simulink model "mechat_taklif2"  (R2016a)
settings: Solver=ode1  StartTime=0.0  StopTime=10.0  FixedStep=0.01  RelTol=1e-3
settings Model: Creator=ALA  LastModifiedBy=ALA

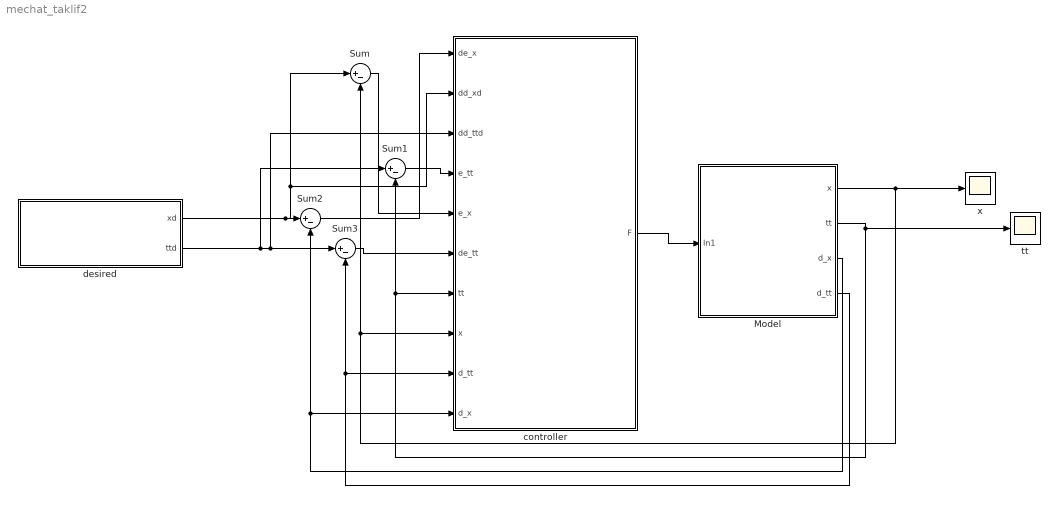
== system mechat_taklif2 ==
  Model : Subsystem
  Sum{,1..3} (4 alike) : Sum  Inputs=|+-
  controller : Subsystem
  desired : Subsystem
  tt : Scope
  x : Scope
  wires:
  controller/1(F) -> Model/1(In1)
  Model/1(x) -> Sum/2, controller/8(x), x/1
  desired/1(xd) -> controller/2(dd_xd), Sum/1, Sum2/1
  desired/2(ttd) -> controller/3(dd_ttd), Sum3/1, Sum1/1
  Model/4(d_tt) -> Sum3/2, controller/9(d_tt)
  Sum/1 -> controller/5("e_x ")
  Sum1/1 -> controller/4("e_tt ")
  Sum2/1 -> controller/1(de_x)
  Sum3/1 -> controller/6(de_tt)
  Model/2(tt) -> Sum1/2, controller/7("tt "), tt/1
  Model/3(d_x) -> Sum2/2, controller/10(d_x)

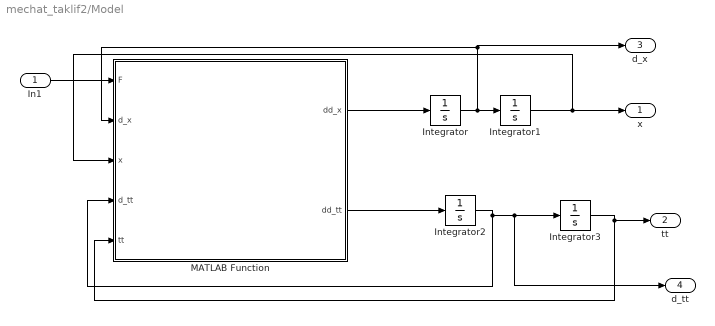
== system mechat_taklif2/Model ==
  In1 : Inport
  Integrator : Integrator
  Integrator1 : Integrator
  Integrator2 : Integrator
  Integrator3 : Integrator  InitialCondition=0.1
  MATLAB Function : MATLAB Function  TreatAsAtomicUnit=on
  x : Outport
  tt : Outport  Port=2
  d_x : Outport  Port=3
  d_tt : Outport  Port=4
  wires:
  In1/1 -> MATLAB Function/1(F)
  MATLAB Function/1(dd_x) -> Integrator/1
  Integrator/1 -> d_x/1, MATLAB Function/2(d_x), Integrator1/1
  Integrator1/1 -> x/1, MATLAB Function/3(x)
  Integrator2/1 -> MATLAB Function/4(d_tt), d_tt/1, Integrator3/1
  Integrator3/1 -> tt/1, MATLAB Function/5(tt)
  MATLAB Function/2(dd_tt) -> Integrator2/1

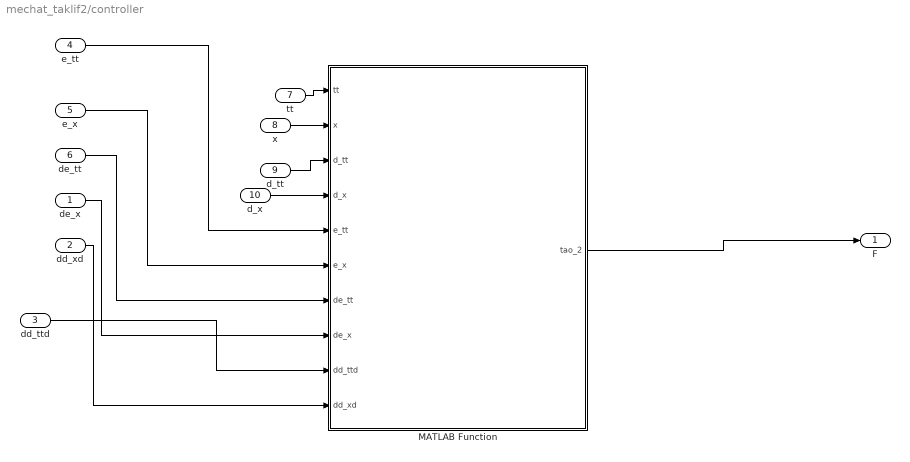
== system mechat_taklif2/controller ==
  de_x : Inport
  dd_xd : Inport  Port=2
  dd_ttd : Inport  Port=3
  "e_tt " : Inport  Port=4
  "e_x " : Inport  Port=5
  de_tt : Inport  Port=6
  "tt " : Inport  Port=7
  x : Inport  Port=8
  d_tt : Inport  Port=9
  d_x : Inport  Port=10
  MATLAB Function : MATLAB Function  TreatAsAtomicUnit=on
  F : Outport
  wires:
  "e_tt "/1 -> MATLAB Function/5(e_tt)
  "e_x "/1 -> MATLAB Function/6(e_x)
  de_tt/1 -> MATLAB Function/7(de_tt)
  de_x/1 -> MATLAB Function/8(de_x)
  dd_xd/1 -> MATLAB Function/10(dd_xd)
  dd_ttd/1 -> MATLAB Function/9(dd_ttd)
  "tt "/1 -> MATLAB Function/1(tt)
  x/1 -> MATLAB Function/2(x)
  d_tt/1 -> MATLAB Function/3(d_tt)
  d_x/1 -> MATLAB Function/4(d_x)
  MATLAB Function/1(tao_2) -> F/1

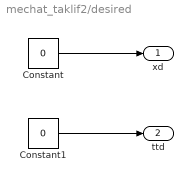
== system mechat_taklif2/desired ==
  Constant : Constant  Value=0
  Constant1 : Constant  Value=0
  xd : Outport
  ttd : Outport  Port=2
  wires:
  Constant/1 -> xd/1
  Constant1/1 -> ttd/1

== matlab function mechat_taklif2/controller/MATLAB Function ==
  data: tt input; x input; d_tt input; d_x input; e_tt input; e_x input; de_tt input; de_x input; dd_ttd input; dd_xd input; tao_2 output
function tao_2 = fcn(tt,x,d_tt,d_x,e_tt,e_x,de_tt,de_x,dd_ttd,dd_xd)
%--------------controller system design-----------------
% 
%           inverted pendulum 
%          (c)copyright 2020,Isfahan University of Technology
%           all rights reserved
% file:
% By:Ala Bazazzadeh   student No.:9638403
% version:
% description:
%-----------------------------------
%-------------------------------

%----------------variables---------------
M = 1; 
m = 1;
L = 1;l = 0.5;g= 9.8;
kp= 150;kd= 300;I= 0;
%------------------------------------------
M_matrix =[I+m*(l^2) m*l*(cos(tt));m*l*(cos(tt)) M+m];

V=[0; -m*l*(d_tt^2)*sin(tt)];
G=[-m*g*l*sin(tt);0];

dd_qd=[dd_ttd;dd_xd];

%------------------e derivatives------------------------
e = [e_tt;e_x];
d_e = [de_tt;de_x];

%-------------------------------------------

tao= M *(dd_qd - kd.*d_e - kp.*e)+V+G;
tao_2=tao(2);

== matlab function mechat_taklif2/Model/MATLAB Function ==
  data: F input; dd_x output; d_x input; x input; d_tt input; tt input; dd_tt output
%------------model------------------
%           inverted pendulum 
%          (c)copyright 2020,Isfahan University of Technology
%           all rights reserved
% file:
% By:Ala Bazazzadeh   student No.:9638403
% version:
% description:
%-----------------------------------

function [dd_x,dd_tt] = model(F,d_x,x,d_tt,tt)
%----------------variables---------------
M = 1; 
m = 1;
L = 1;
l = 0.5;
g = 9.8;
I=0;
%----------------Dynamic equations-------
M_matrix=[I+m*(l^2) m*l*(cos(tt));m*l*(cos(tt)) M+m];
V=[0; -m*l*(d_tt^2)*sin(tt)];
G=[-m*g*l*sin(tt);0];

ta = [0;F];

q=inv(M_matrix) * (ta - V - G);
dd_tt = q(1);
dd_x = q(2);
